simulink model "Earth_position"  (R2023b)
settings: Solver=FixedStepAuto  StartTime=0.0  StopTime=36525/2  FixedStep=1/24  RelTol=1/24
libraries: vrlib x2, nav_lib x1, aerolibconvert2 x1, simulink_extras x1
settings Model: DataDictionary=Navigation.sldd  Creator=brent  LastModifiedBy=brent

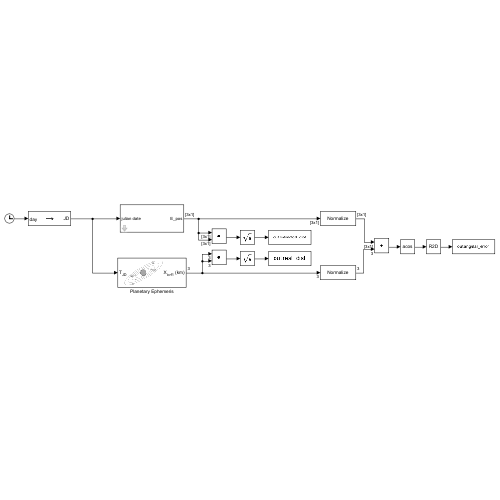
[thumbnail: Simulink's stored preview of the top-level diagram]
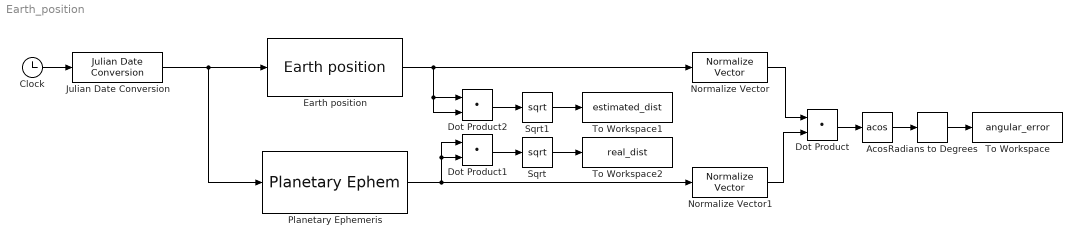
== system Earth_position ==
  Acos : Trigonometry  Operator=acos
  Clock : Clock
  Dot Product : DotProduct  OutDataTypeStr=Inherit: Inherit via internal rule
  Dot Product1 : DotProduct  OutDataTypeStr=Inherit: Inherit via internal rule
  Dot Product2 : DotProduct  OutDataTypeStr=Inherit: Inherit via internal rule
  Earth position : nav_lib/Earth position  amp=Propagation.Earth.amp.value  freq=Propagation.Earth.freq.value  phase=Propagation.Earth.phase.value
      settings: SourceProductName=Navigation library
  Julian Date Conversion : aerolibconvert2/Julian Date Conversion  year=2000  month=January  day=1  hour=12  min=0  sec=0  modflag=off  deltaT=Day  errorflag=Error
  Normalize Vector : vrlib/Utilities/Normalize Vector  maxzero=0
  Normalize Vector1 : vrlib/Utilities/Normalize Vector  maxzero=0
  Planetary Ephemeris : PlanetaryEphem  center=Moon  target=Earth  outputVelocity=off
  Radians to Degrees : simulink_extras/Transformations/Radians to Degrees
  Sqrt : Sqrt
  Sqrt1 : Sqrt
  To Workspace : ToWorkspace  VariableName=angular_error  SampleTime=-1
      settings: Save2DSignal=2-D array (concatenate along first dimension)
  To Workspace1 : ToWorkspace  VariableName=estimated_dist  SampleTime=-1
      settings: Save2DSignal=2-D array (concatenate along first dimension)
  To Workspace2 : ToWorkspace  VariableName=real_dist  SampleTime=-1
      settings: Save2DSignal=2-D array (concatenate along first dimension)
  wires:
  Clock/1 -> Julian Date Conversion/1
  Julian Date Conversion/1 -> Planetary Ephemeris/1, Earth position/1
  Planetary Ephemeris/1 -> Dot Product1/1, Dot Product1/2, Normalize Vector1/1
  Normalize Vector1/1 -> Dot Product/2
  Normalize Vector/1 -> Dot Product/1
  Dot Product/1 -> Acos/1
  Acos/1 -> Radians to Degrees/1
  Radians to Degrees/1 -> To Workspace/1
  Earth position/1 -> Dot Product2/2, Dot Product2/1, Normalize Vector/1
  Dot Product1/1 -> Sqrt/1
  Dot Product2/1 -> Sqrt1/1
  Sqrt1/1 -> To Workspace1/1
  Sqrt/1 -> To Workspace2/1
